simulink model "planetary_gearbox"  (R2023a)
settings: Solver=VariableStepAuto  StartTime=0.0  StopTime=10.0  RelTol=1e-3
undefined symbols (not defined in the file): i_pgb
settings Model: Creator=Artem Sannikov  LastModifiedBy=Artem Sannikov

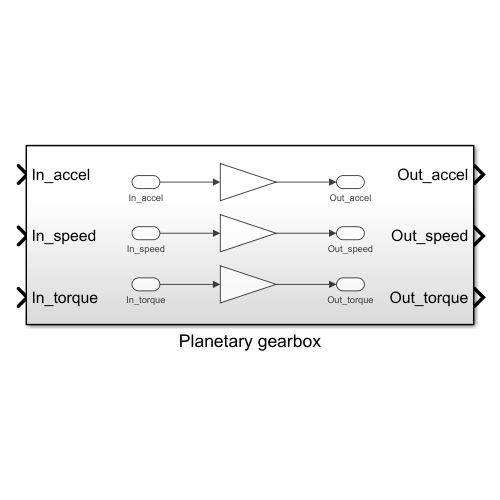
[thumbnail: Simulink's stored preview of the top-level diagram]
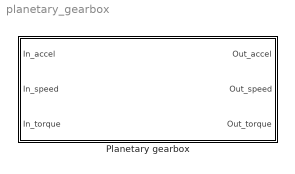
== system planetary_gearbox ==
  Planetary gearbox : Subsystem

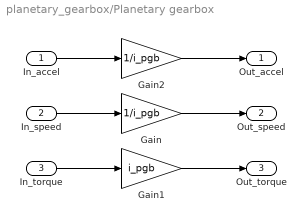
== system planetary_gearbox/Planetary gearbox ==
  In_accel : Inport
  In_speed : Inport  Port=2
  In_torque : Inport  Port=3
  Gain : Gain  Gain=1/i_pgb
  Gain1 : Gain  Gain=i_pgb
  Gain2 : Gain  Gain=1/i_pgb
  Out_accel : Outport
  Out_speed : Outport  Port=2
  Out_torque : Outport  Port=3
  wires:
  In_speed/1 -> Gain/1
  Gain/1 -> Out_speed/1
  In_torque/1 -> Gain1/1
  Gain1/1 -> Out_torque/1
  In_accel/1 -> Gain2/1
  Gain2/1 -> Out_accel/1
